simulink model "boost_converter_mppt"  (R2023a)
settings: Solver=VariableStepAuto  StartTime=0.0  StopTime=10.0  RelTol=1e-3
PreLoadFcn:
  | Ts_Power=50e-6;
  | Ts_Control=100e-6;
libraries: spsSeriesRLCBranchLib x4, spsCurrentMeasurementLib x1, spsDiodeLib x1, spsStairGeneratorLib x1, spsPWMGeneratorDCDCLib x1, spsPVArrayLib x1, spsIGBTDiodeLib x1, spsVoltageMeasurementLib x1, sps_lib x1
settings Model: Creator=hp  LastModifiedBy=hp

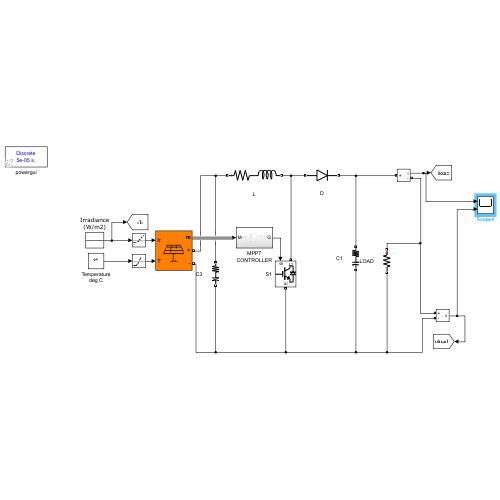
[thumbnail: Simulink's stored preview of the top-level diagram]
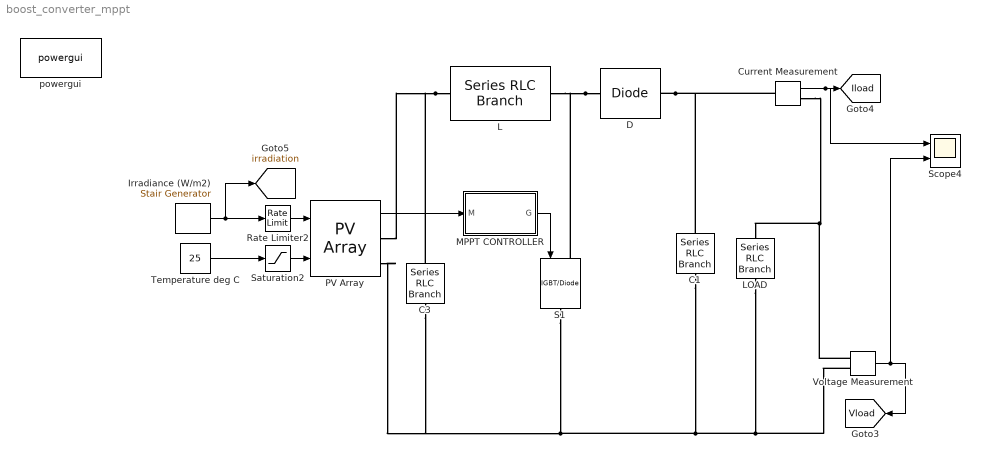
== system boost_converter_mppt ==
  C1 : spsSeriesRLCBranchLib/Series RLC Branch  LConnTagsString=__new0  RConnTagsString=__new0  BranchType=RC  Resistance=0.001  Inductance=1e-3  SetiL0=off  InitialCurrent=0  Capacitance=16000e-6  Setx0=off  InitialVoltage=350  Measurements=None
  C3 : spsSeriesRLCBranchLib/Series RLC Branch  LConnTagsString=__new0  RConnTagsString=__new0  BranchType=RC  Resistance=0.0001  Inductance=1e-3  SetiL0=off  InitialCurrent=0  Capacitance=220e-6  Setx0=off  InitialVoltage=350  Measurements=None
  Current Measurement : spsCurrentMeasurementLib/Current Measurement  PhasorSimulation=off  OutputType=Complex  PSBequivalent=0
  D : spsDiodeLib/Diode  Ron=0.001  Lon=0  Vf=0.8  IC=0  UseSnubber=0  Rs=inf  Cs=250e-9  Measurements=off
  Irradiance (W/m2) : spsStairGeneratorLib/Stair Generator  t=[0 2.5 4.5 8.5 10]  e=[900 900 900 900 900]  Ts=50e-6
  L : spsSeriesRLCBranchLib/Series RLC Branch  LConnTagsString=__new0  RConnTagsString=__new0  BranchType=RL  Resistance=0.001  Inductance=4e-3  SetiL0=off  InitialCurrent=0  Capacitance=1e-6  Setx0=off  InitialVoltage=0  Measurements=None
  LOAD : spsSeriesRLCBranchLib/Series RLC Branch  LConnTagsString=__new0  RConnTagsString=__new0  BranchType=R  Resistance=5  Inductance=1e-3  SetiL0=off  InitialCurrent=0  Capacitance=4700e-6  Setx0=on  InitialVoltage=350  Measurements=None
  MPPT CONTROLLER : Subsystem
  PV Array : spsPVArrayLib/PV Array  Npar=9.5  Nser=0.396  PlotType=array @ 1000 W/m2 & specified temperatures  S_vec="[ 1000  500  100 ]"  Temp_C_vec="[ 45 25  ]"  ModuleName=SunPower SPR-315E-WHT-D  PlotWhenSelected=off  Pm=315.072  Ncell=96  Voc=64.6  Isc=6.14  Vm=54.7  Im=5.76  beta_Voc_pc=-0.2727  alpha_Isc_pc=0.061743  beta_Voc=-0.17616  alpha_Isc=0.003791  IL=6.1461  I0=6.5067e-12  nI=0.95071  Rsh=430.0666  Rs=0.43041  RobustModel=off  RobustCellTemperature=313.3991  BAL=off  Tc=1e-6  Tfilter=5e-5
  Rate Limiter2 : RateLimiter  RisingSlewLimit=8000  FallingSlewLimit=-8000  SampleTimeMode=inherited  InitialCondition=1000
  S1 : spsIGBTDiodeLib/IGBT//Diode  Ron=1e-3  Rs=1e5  Cs=inf  Measurements=off
  Saturation2 : Saturate  UpperLimit=55  LowerLimit=5
  Scope4 : Scope  NumInputPorts=2
  Temperature deg C : Constant  Value=25
  Voltage Measurement : spsVoltageMeasurementLib/Voltage Measurement  PhasorSimulation=off  OutputType=Complex  PSBequivalent=0
  powergui : sps_lib/powergui  Priority=1  SimulationMode=Discrete  SampleTime=50e-6  frequency=60  Iterations=50  frequencyindice=0  Pbase=100e6  ErrMax=1e-4  UnitsV=kV  UnitsW=MW  buscounter=0  FunctionMessages=off  echomessages=off  EnableUseOfTLC=off  CurrentSourceSwitches=off  DisableSnubberDevices=off  DisableRonSwitches=off  DisableVfSwitches=off  DisplayEquations=off  AutomaticDiscreteSolvers=off  SolverType=Tustin/Backward Euler (TBE)  Interpol=off  ExternalGateDelay=off  methode=off  Ts=100  x0status=blocks  SPID=on  SwTol=0  HookPort=off  NonlinearTolerance=1e-4  nMaxIteration=100  ContinueOnMaxIteration=off  RestoreLinks=warning  ResistiveCurrentMeasurement=off  Frange=[0:2:500]  Ylog=off  Xlog=on  ShowGrid=off  save=off  variable=ZData  structure=0  ZoomFFT=off  StartTime=0.0  cycles=1  DisplayStyle=1  fundamental=60  FreqAxis=off  MaxFrequency=1000  frequencyindicesteady=1  RmsSteady=1  display=off
  tag scope: Iload=global, Vload=global, irradiation=global
  wires:
  MPPT CONTROLLER/1(G) -> S1/1
  Voltage Measurement/1 -> Scope4/2, [Vload]
  Rate Limiter2/1 -> PV Array/1
  Saturation2/1 -> PV Array/2
  Current Measurement/1 -> Scope4/1, [Iload]
  Irradiance (W/m2)/1 -> [irradiation], Rate Limiter2/1
  PV Array/1 -> MPPT CONTROLLER/1(M)
  Temperature deg C/1 -> Saturation2/1
  connections:
  D/RConn1 -- Current Measurement/LConn1 -- C1/LConn1
  LOAD/RConn1 -- Voltage Measurement/LConn2 -- PV Array/RConn2 -- C3/RConn1 -- S1/RConn1 -- C1/RConn1
  D/LConn1 -- L/RConn1 -- S1/LConn1
  Current Measurement/RConn1 -- Voltage Measurement/LConn1 -- LOAD/LConn1
  L/LConn1 -- C3/LConn1 -- PV Array/RConn1

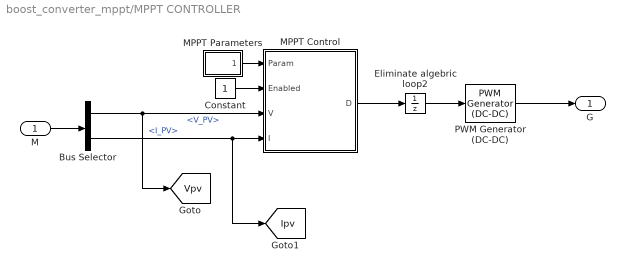
== system boost_converter_mppt/MPPT CONTROLLER ==
  M : Inport
  Bus Selector : BusSelector  OutputSignals=V_PV,I_PV
  Constant : Constant
  Eliminate algebric loop2 : UnitDelay  InitialCondition=0.485  SampleTime=Ts_Control  HasFrameUpgradeWarning=on
  MPPT Parameters : Subsystem
  "MPPT Control  " : MATLAB Function  TreatAsAtomicUnit=on
  PWM Generator (DC-DC) : spsPWMGeneratorDCDCLib/PWM Generator (DC-DC)  Fsw=5000  Ts=50e-6
  G : Outport  VectorParamsAs1DForOutWhenUnconnected=off
  tag scope: Ipv=global, Vpv=global
  wires:
  Bus Selector/2 -> [Ipv], "MPPT Control  "/4(I)  "<I_PV>"
  M/1 -> Bus Selector/1
  "MPPT Control  "/1(D) -> Eliminate algebric loop2/1
  Constant/1 -> "MPPT Control  "/2(Enabled)
  Bus Selector/1 -> [Vpv], "MPPT Control  "/3(V)  "<V_PV>"
  Eliminate algebric loop2/1 -> PWM Generator (DC-DC)/1
  MPPT Parameters/1(Param) -> "MPPT Control  "/1(Param)
  PWM Generator (DC-DC)/1 -> G/1

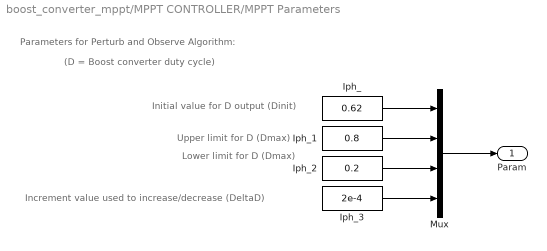
== system boost_converter_mppt/MPPT CONTROLLER/MPPT Parameters ==
  note: Upper limit for D (Dmax)
  note: Increment value used to increase/decrease (DeltaD)
  note: Initial value for D output (Dinit)
  note: (D = Boost converter duty cycle)
  note: Lower limit for D (Dmax)
  note: Parameters for Perturb and Observe Algorithm:
  Iph_ : Constant  Value=0.62
  Iph_1 : Constant  Value=0.8
  Iph_2 : Constant  Value=0.2
  Iph_3 : Constant  Value=2e-4
  Mux : Mux
  Param : Outport  VectorParamsAs1DForOutWhenUnconnected=off
  wires:
  Iph_/1 -> Mux/1
  Iph_1/1 -> Mux/2
  Iph_2/1 -> Mux/3
  Iph_3/1 -> Mux/4
  Mux/1 -> Param/1

== matlab function boost_converter_mppt/MPPT CONTROLLER/MPPT Control   ==
  settings: updateMethod=DISCRETE  sampleTime=Ts_Control
  data: Param input; Enabled input; V input =V; I input; D output
function D  = PandO(Param, Enabled, V, I)

% MPPT controller based on the Perturb & Observe algorithm.

% D output = Duty cycle of the boost converter (value between 0 and 1)
%
% Enabled input = 1 to enable the MPPT controller
% V input = PV array terminal voltage (V)
% I input = PV array current (A)
%
% Param input:
Dinit = Param(1);  %Initial value for D output
Dmax = Param(2);   %Maximum value for D
Dmin = Param(3);   %Minimum value for D
deltaD = Param(4); %Increment value used to increase/decrease the duty cycle D
% ( increasing D = decreasing Vref )
%  

persistent Vold Pold Dold;

dataType = 'double';

if isempty(Vold)
    Vold=0;
    Pold=0;
    Dold=Dinit;
end
P= V*I;
dV= V - Vold;
dP= P - Pold;

if dP ~= 0 & Enabled ~=0
    if dP < 0
        if dV < 0
            D = Dold - deltaD;
        else
            D = Dold + deltaD;
        end
    else
        if dV < 0
            D = Dold + deltaD;
        else
            D = Dold - deltaD;
        end    
    end
else D=Dold;
end

if D >= Dmax | D<= Dmin
    D=Dold;
end

Dold=D;
Vold=V;
Pold=P;
